simulink model "vocoder_model"  (R2017b)
settings: Solver=VariableStepAuto  StartTime=0.0  StopTime=20  RelTol=1e-3
undefined symbols (not defined in the file or in its folder): NB
libraries: xbsIndex_r4 x1026, dspsrcs4 x1
(part 1 of 8)
settings Model: Creator=8183302  LastModifiedBy=8183302

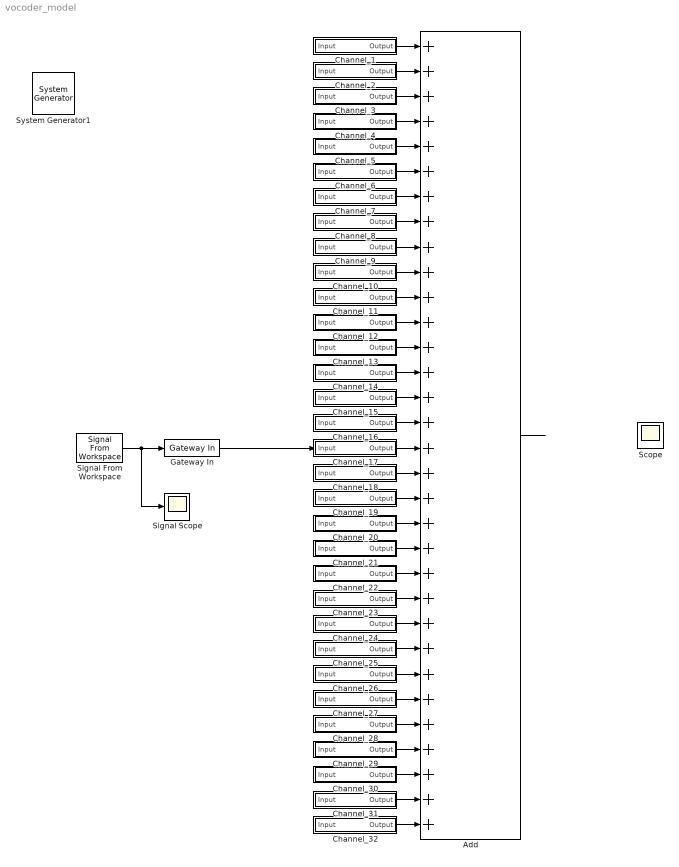
== system vocoder_model ==
  " System Generator1" : xbsIndex_r4/ System Generator  Tag=genX  xilinxfamily=kintex7  part=xc7k325t  speed=-3  package=fbg676  synthesis_tool=Vivado  clock_wrapper=Clock Enables  directory=./netlist  proj_type=Vivado  Synth_file=Vivado Synthesis Defaults  Impl_file=Vivado Implementation Defaults  testbench=off  simulink_period=1/8000  sysclk_period=10  dcm_input_clock_period=10  incr_netlist=off  trim_vbits=Everywhere in SubSystem  dbl_ovrd=According to Block Masks  core_generation=According to Block Masks  run_coregen=off  deprecated_control=off  eval_field=0  block_type=sysgen
  Add : Sum  Inputs=++++++++++++++++++++++++++++++++
  Channel_1 : Subsystem  mask{b0=0.1426970149, b1=0.0000000000, b2=-0.1426970149, a1=-1.6901715989, a2=0.7146059702, fc=299.991723}
  Channel_10 : Subsystem  mask{b0=0.0872963307, b1=0.0000000000, b2=-0.0872963307, a1=-1.4690457093, a2=0.8254073387, fc=816.949484}
  Channel_11 : Subsystem  mask{b0=0.0845435910, b1=0.0000000000, b2=-0.0845435910, a1=-1.4085768543, a2=0.8309128181, fc=888.837275}
  Channel_12 : Subsystem  mask{b0=0.0820880005, b1=0.0000000000, b2=-0.0820880005, a1=-1.3394973368, a2=0.8358239989, fc=964.131808}
  Channel_13 : Subsystem  mask{b0=0.0798861132, b1=0.0000000000, b2=-0.0798861132, a1=-1.2612912570, a2=0.8402277736, fc=1042.994526}
  Channel_14 : Subsystem  mask{b0=0.0779025394, b1=0.0000000000, b2=-0.0779025394, a1=-1.1734445637, a2=0.8441949212, fc=1125.594525}
  Channel_15 : Subsystem  mask{b0=0.0761081589, b1=0.0000000000, b2=-0.0761081589, a1=-1.0754648676, a2=0.8477836822, fc=1212.108914}
  Channel_16 : Subsystem  mask{b0=0.0744787896, b1=0.0000000000, b2=-0.0744787896, a1=-0.9669048108, a2=0.8510424209, fc=1302.723195}
  Channel_17 : Subsystem  mask{b0=0.0729941817, b1=0.0000000000, b2=-0.0729941817, a1=-0.8473898380, a2=0.8540116366, fc=1397.631659}
  Channel_18 : Subsystem  mask{b0=0.0716372491, b1=0.0000000000, b2=-0.0716372491, a1=-0.7166511718, a2=0.8567255018, fc=1497.037808}
  Channel_19 : Subsystem  mask{b0=0.0703934733, b1=0.0000000000, b2=-0.0703934733, a1=-0.5745647402, a2=0.8592130535, fc=1601.154785}
  Channel_2 : Subsystem  mask{b0=0.1312430755, b1=0.0000000000, b2=-0.1312430755, a1=-1.6922316836, a2=0.7375138489, fc=347.381037}
  Channel_20 : Subsystem  mask{b0=0.0692504382, b1=0.0000000000, b2=-0.0692504382, a1=-0.4211967011, a2=0.8614991237, fc=1710.205836}
  Channel_21 : Subsystem  mask{b0=0.0681974623, b1=0.0000000000, b2=-0.0681974623, a1=-0.2568560434, a2=0.8636050755, fc=1824.424783}
  Channel_22 : Subsystem  mask{b0=0.0672253054, b1=0.0000000000, b2=-0.0672253054, a1=-0.0821544768, a2=0.8655493893, fc=1944.056533}
  Channel_23 : Subsystem  mask{b0=0.0663259331, b1=0.0000000000, b2=-0.0663259331, a1=0.1019265783, a2=0.8673481338, fc=2069.357596}
  Channel_24 : Subsystem  mask{b0=0.0654923262, b1=0.0000000000, b2=-0.0654923262, a1=0.2939626743, a2=0.8690153475, fc=2200.596640}
  Channel_25 : Subsystem  mask{b0=0.0647183248, b1=0.0000000000, b2=-0.0647183248, a1=0.4920082741, a2=0.8705633504, fc=2338.055064}
  Channel_26 : Subsystem  mask{b0=0.0639985006, b1=0.0000000000, b2=-0.0639985006, a1=0.6935166168, a2=0.8720029989, fc=2482.027602}
  Channel_27 : Subsystem  mask{b0=0.0633280511, b1=0.0000000000, b2=-0.0633280511, a1=0.8952616127, a2=0.8733438978, fc=2632.822957}
  Channel_28 : Subsystem  mask{b0=0.0627027123, b1=0.0000000000, b2=-0.0627027123, a1=1.0932676802, a2=0.8745945754, fc=2790.764459}
  Channel_29 : Subsystem  mask{b0=0.0621186846, b1=0.0000000000, b2=-0.0621186846, a1=1.2827556587, a2=0.8757626308, fc=2956.190763}
  Channel_3 : Subsystem  mask{b0=0.1219971552, b1=0.0000000000, b2=-0.1219971552, a1=-1.6873845160, a2=0.7560056896, fc=397.016117}
  Channel_30 : Subsystem  mask{b0=0.0615725716, b1=0.0000000000, b2=-0.0615725716, a1=1.4581155660, a2=0.8768548568, fc=3129.456570}
  Channel_31 : Subsystem  mask{b0=0.0610613278, b1=0.0000000000, b2=-0.0610613278, a1=1.6129199398, a2=0.8778773445, fc=3310.933394}
  Channel_32 : Subsystem  mask{b0=0.0605822143, b1=0.0000000000, b2=-0.0605822143, a1=1.7399946660, a2=0.8788355715, fc=3501.010351}
  Channel_4 : Subsystem  mask{b0=0.1143823509, b1=0.0000000000, b2=-0.1143823509, a1=-1.6760436191, a2=0.7712352982, fc=449.003389}
  Channel_5 : Subsystem  mask{b0=0.1080071943, b1=0.0000000000, b2=-0.1080071943, a1=-1.6583545791, a2=0.7839856114, fc=503.454323}
  Channel_6 : Subsystem  mask{b0=0.1025964806, b1=0.0000000000, b2=-0.1025964806, a1=-1.6342751055, a2=0.7948070389, fc=560.485670}
  Channel_7 : Subsystem  mask{b0=0.0979509870, b1=0.0000000000, b2=-0.0979509870, a1=-1.6036256537, a2=0.8040980260, fc=620.219716}
  Channel_8 : Subsystem  mask{b0=0.0939228891, b1=0.0000000000, b2=-0.0939228891, a1=-1.5661230792, a2=0.8121542217, fc=682.784541}
  Channel_9 : Subsystem  mask{b0=0.0904001591, b1=0.0000000000, b2=-0.0904001591, a1=-1.5214045021, a2=0.8191996818, fc=748.314295}
  Gateway In : xbsIndex_r4/Gateway In  gui_display_data_type=Fixed-point  arith_type="Signed  (2's comp)"  n_bits=16  bin_pt=15  preci_type=Single  exp_width=8  frac_width=24  rows=1  columns=1  quantization="Round  (unbiased: +/- Inf)"  overflow=Saturate  period=1/8000  UseAsADC=off  ADCChannel='1'  interface=None  automatic_assignment=on  address_offset=hex2dec('00')  intf_name=''  intf_description=''  default_value=0  timing_constraint=None  locs_specified=off  LOCs={}  io_standard={}  inherit_from_input=off  hdl_port=on  dbl_ovrd=off  block_type=gatewayin
  Scope : Scope
  Signal From Workspace : dspsrcs4/Signal From Workspace  X=x  Ts=1/8000  nsamps=1  OutputAfterFinalValue=Setting to zero  ignoreOrWarnInputAndFrameLengths=off  OutputFrames=off
  Signal Scope : Scope
  wires:
  Signal From Workspace/1 -> Signal Scope/1, Gateway In/1
  Channel_1/1(Output) -> Add/1
  Channel_2/1(Output) -> Add/2
  Channel_3/1(Output) -> Add/3
  Channel_4/1(Output) -> Add/4
  Channel_5/1(Output) -> Add/5
  Channel_6/1(Output) -> Add/6
  Channel_7/1(Output) -> Add/7
  Channel_8/1(Output) -> Add/8
  Channel_9/1(Output) -> Add/9
  Channel_10/1(Output) -> Add/10
  Channel_11/1(Output) -> Add/11
  Channel_12/1(Output) -> Add/12
  Channel_13/1(Output) -> Add/13
  Channel_14/1(Output) -> Add/14
  Channel_15/1(Output) -> Add/15
  Channel_16/1(Output) -> Add/16
  Channel_17/1(Output) -> Add/17
  Channel_18/1(Output) -> Add/18
  Channel_19/1(Output) -> Add/19
  Channel_20/1(Output) -> Add/20
  Channel_21/1(Output) -> Add/21
  Channel_22/1(Output) -> Add/22
  Channel_23/1(Output) -> Add/23
  Channel_24/1(Output) -> Add/24
  Channel_25/1(Output) -> Add/25
  Channel_26/1(Output) -> Add/26
  Channel_27/1(Output) -> Add/27
  Channel_28/1(Output) -> Add/28
  Channel_29/1(Output) -> Add/29
  Channel_30/1(Output) -> Add/30
  Channel_31/1(Output) -> Add/31
  Channel_32/1(Output) -> Add/32
  Add/1 -> ?
  Gateway In/1 -> Channel_17/1(Input)
  ? -> Scope/1

== system vocoder_model/Channel_1 ==
  Input : Inport
  Abs Scope : Scope
  Absolute : xbsIndex_r4/Absolute  precision=User Defined  arith_type="Signed  (2's comp)"  n_bits=16  bin_pt=15  quantization=Truncate  overflow=Wrap  en=off  latency=0  dbl_ovrd=off  block_type=abs
  Convert : xbsIndex_r4/Convert  gui_display_data_type=Fixed-point  arith_type="Signed  (2's comp)"  n_bits=16  bin_pt=15  float_type=Single  exp_bits=8  fraction_bits=24  quantization=Truncate  overflow=Wrap  en=off  latency=0  pipeline=off  dbl_ovrd=off  block_type=convert
  Final Channel Scope : Scope
  Gateway In : xbsIndex_r4/Gateway In  gui_display_data_type=Fixed-point  arith_type="Signed  (2's comp)"  n_bits=16  bin_pt=15  preci_type=Single  exp_width=8  frac_width=24  rows=1  columns=1  quantization=Truncate  overflow=Wrap  period=1/8000  UseAsADC=off  ADCChannel='1'  interface=None  automatic_assignment=on  address_offset=hex2dec('00')  intf_name=''  intf_description=''  default_value=0  timing_constraint=None  locs_specified=off  LOCs={}  io_standard={}  inherit_from_input=off  hdl_port=on  dbl_ovrd=off  block_type=gatewayin
  Gateway Out{,1..3} (4 alike) : xbsIndex_r4/Gateway Out  inherit_from_input=off  hdl_port=off  rows=1  columns=1  UseAsDAC=off  DACChannel='1'  interface=None  automatic_assignment=on  address_offset=hex2dec('00')  intf_name=''  intf_description=''  timing_constraint=None  locs_specified=off  LOCs={}  io_standard={}  block_type=gatewayout
  IIR Filter : Subsystem
  IIR Filter Scope : Scope
  LPF Scope : Scope
  Low Pass Filter : Subsystem
  Mult : xbsIndex_r4/Mult  precision=User Defined  arith_type="Signed  (2's comp)"  n_bits=16  bin_pt=15  quantization=Truncate  overflow=Wrap  en=off  latency=0  use_behavioral_HDL=off  opt=Speed  use_embedded=on  optimum_pipeline=off  pipeline=on  dbl_ovrd=off  use_rpm=on  placement_style=Triangular  block_type=mult
  Sine Wave : Sin  Frequency=2*pi*fc  SampleTime=1/8000
  Output : Outport
  wires:
  Input/1 -> IIR Filter/1(Input)
  IIR Filter/1(Output) -> Gateway Out1/1, Absolute/1
  Sine Wave/1 -> Gateway In/1
  Convert/1 -> Mult/1
  Gateway In/1 -> Mult/2
  Absolute/1 -> Gateway Out2/1, Low Pass Filter/1(Input1)
  Low Pass Filter/1(Output1) -> Gateway Out3/1, Convert/1
  Gateway Out/1 -> Output/1, Final Channel Scope/1
  Mult/1 -> Gateway Out/1
  Gateway Out1/1 -> IIR Filter Scope/1
  Gateway Out2/1 -> Abs Scope/1
  Gateway Out3/1 -> LPF Scope/1

== system vocoder_model/Channel_10 ==
  Input : Inport
  Abs Scope : Scope
  Absolute : xbsIndex_r4/Absolute  precision=User Defined  arith_type="Signed  (2's comp)"  n_bits=16  bin_pt=15  quantization=Truncate  overflow=Wrap  en=off  latency=0  dbl_ovrd=off  block_type=abs
  Convert : xbsIndex_r4/Convert  gui_display_data_type=Fixed-point  arith_type="Signed  (2's comp)"  n_bits=16  bin_pt=15  float_type=Single  exp_bits=8  fraction_bits=24  quantization=Truncate  overflow=Wrap  en=off  latency=0  pipeline=off  dbl_ovrd=off  block_type=convert
  Final Channel Scope : Scope
  Gateway In : xbsIndex_r4/Gateway In  gui_display_data_type=Fixed-point  arith_type="Signed  (2's comp)"  n_bits=16  bin_pt=15  preci_type=Single  exp_width=8  frac_width=24  rows=1  columns=1  quantization=Truncate  overflow=Wrap  period=1/8000  UseAsADC=off  ADCChannel='1'  interface=None  automatic_assignment=on  address_offset=hex2dec('00')  intf_name=''  intf_description=''  default_value=0  timing_constraint=None  locs_specified=off  LOCs={}  io_standard={}  inherit_from_input=off  hdl_port=on  dbl_ovrd=off  block_type=gatewayin
  Gateway Out{,1..3} (4 alike) : xbsIndex_r4/Gateway Out  inherit_from_input=off  hdl_port=off  rows=1  columns=1  UseAsDAC=off  DACChannel='1'  interface=None  automatic_assignment=on  address_offset=hex2dec('00')  intf_name=''  intf_description=''  timing_constraint=None  locs_specified=off  LOCs={}  io_standard={}  block_type=gatewayout
  IIR Filter : Subsystem
  IIR Filter Scope : Scope
  LPF Scope : Scope
  Low Pass Filter : Subsystem
  Mult : xbsIndex_r4/Mult  precision=User Defined  arith_type="Signed  (2's comp)"  n_bits=16  bin_pt=15  quantization=Truncate  overflow=Wrap  en=off  latency=0  use_behavioral_HDL=off  opt=Speed  use_embedded=on  optimum_pipeline=off  pipeline=on  dbl_ovrd=off  use_rpm=on  placement_style=Triangular  block_type=mult
  Sine Wave : Sin  Frequency=2*pi*fc  SampleTime=1/8000
  Output : Outport
  wires:
  Input/1 -> IIR Filter/1(Input)
  IIR Filter/1(Output) -> Gateway Out1/1, Absolute/1
  Sine Wave/1 -> Gateway In/1
  Convert/1 -> Mult/1
  Gateway In/1 -> Mult/2
  Absolute/1 -> Gateway Out2/1, Low Pass Filter/1(Input1)
  Low Pass Filter/1(Output1) -> Gateway Out3/1, Convert/1
  Gateway Out/1 -> Output/1, Final Channel Scope/1
  Mult/1 -> Gateway Out/1
  Gateway Out1/1 -> IIR Filter Scope/1
  Gateway Out2/1 -> Abs Scope/1
  Gateway Out3/1 -> LPF Scope/1

== system vocoder_model/Channel_11 ==
  Input : Inport
  Abs Scope : Scope
  Absolute : xbsIndex_r4/Absolute  precision=User Defined  arith_type="Signed  (2's comp)"  n_bits=16  bin_pt=15  quantization=Truncate  overflow=Wrap  en=off  latency=0  dbl_ovrd=off  block_type=abs
  Convert : xbsIndex_r4/Convert  gui_display_data_type=Fixed-point  arith_type="Signed  (2's comp)"  n_bits=16  bin_pt=15  float_type=Single  exp_bits=8  fraction_bits=24  quantization=Truncate  overflow=Wrap  en=off  latency=0  pipeline=off  dbl_ovrd=off  block_type=convert
  Final Channel Scope : Scope
  Gateway In : xbsIndex_r4/Gateway In  gui_display_data_type=Fixed-point  arith_type="Signed  (2's comp)"  n_bits=16  bin_pt=15  preci_type=Single  exp_width=8  frac_width=24  rows=1  columns=1  quantization=Truncate  overflow=Wrap  period=1/8000  UseAsADC=off  ADCChannel='1'  interface=None  automatic_assignment=on  address_offset=hex2dec('00')  intf_name=''  intf_description=''  default_value=0  timing_constraint=None  locs_specified=off  LOCs={}  io_standard={}  inherit_from_input=off  hdl_port=on  dbl_ovrd=off  block_type=gatewayin
  Gateway Out{,1..3} (4 alike) : xbsIndex_r4/Gateway Out  inherit_from_input=off  hdl_port=off  rows=1  columns=1  UseAsDAC=off  DACChannel='1'  interface=None  automatic_assignment=on  address_offset=hex2dec('00')  intf_name=''  intf_description=''  timing_constraint=None  locs_specified=off  LOCs={}  io_standard={}  block_type=gatewayout
  IIR Filter : Subsystem
  IIR Filter Scope : Scope
  LPF Scope : Scope
  Low Pass Filter : Subsystem
  Mult : xbsIndex_r4/Mult  precision=User Defined  arith_type="Signed  (2's comp)"  n_bits=16  bin_pt=15  quantization=Truncate  overflow=Wrap  en=off  latency=0  use_behavioral_HDL=off  opt=Speed  use_embedded=on  optimum_pipeline=off  pipeline=on  dbl_ovrd=off  use_rpm=on  placement_style=Triangular  block_type=mult
  Sine Wave : Sin  Frequency=2*pi*fc  SampleTime=1/8000
  Output : Outport
  wires:
  Input/1 -> IIR Filter/1(Input)
  IIR Filter/1(Output) -> Gateway Out1/1, Absolute/1
  Sine Wave/1 -> Gateway In/1
  Convert/1 -> Mult/1
  Gateway In/1 -> Mult/2
  Absolute/1 -> Gateway Out2/1, Low Pass Filter/1(Input1)
  Low Pass Filter/1(Output1) -> Gateway Out3/1, Convert/1
  Gateway Out/1 -> Output/1, Final Channel Scope/1
  Mult/1 -> Gateway Out/1
  Gateway Out1/1 -> IIR Filter Scope/1
  Gateway Out2/1 -> Abs Scope/1
  Gateway Out3/1 -> LPF Scope/1

== system vocoder_model/Channel_12 ==
  Input : Inport
  Abs Scope : Scope
  Absolute : xbsIndex_r4/Absolute  precision=User Defined  arith_type="Signed  (2's comp)"  n_bits=16  bin_pt=15  quantization=Truncate  overflow=Wrap  en=off  latency=0  dbl_ovrd=off  block_type=abs
  Convert : xbsIndex_r4/Convert  gui_display_data_type=Fixed-point  arith_type="Signed  (2's comp)"  n_bits=16  bin_pt=15  float_type=Single  exp_bits=8  fraction_bits=24  quantization=Truncate  overflow=Wrap  en=off  latency=0  pipeline=off  dbl_ovrd=off  block_type=convert
  Final Channel Scope : Scope
  Gateway In : xbsIndex_r4/Gateway In  gui_display_data_type=Fixed-point  arith_type="Signed  (2's comp)"  n_bits=16  bin_pt=15  preci_type=Single  exp_width=8  frac_width=24  rows=1  columns=1  quantization=Truncate  overflow=Wrap  period=1/8000  UseAsADC=off  ADCChannel='1'  interface=None  automatic_assignment=on  address_offset=hex2dec('00')  intf_name=''  intf_description=''  default_value=0  timing_constraint=None  locs_specified=off  LOCs={}  io_standard={}  inherit_from_input=off  hdl_port=on  dbl_ovrd=off  block_type=gatewayin
  Gateway Out{,1..3} (4 alike) : xbsIndex_r4/Gateway Out  inherit_from_input=off  hdl_port=off  rows=1  columns=1  UseAsDAC=off  DACChannel='1'  interface=None  automatic_assignment=on  address_offset=hex2dec('00')  intf_name=''  intf_description=''  timing_constraint=None  locs_specified=off  LOCs={}  io_standard={}  block_type=gatewayout
  IIR Filter : Subsystem
  IIR Filter Scope : Scope
  LPF Scope : Scope
  Low Pass Filter : Subsystem
  Mult : xbsIndex_r4/Mult  precision=User Defined  arith_type="Signed  (2's comp)"  n_bits=16  bin_pt=15  quantization=Truncate  overflow=Wrap  en=off  latency=0  use_behavioral_HDL=off  opt=Speed  use_embedded=on  optimum_pipeline=off  pipeline=on  dbl_ovrd=off  use_rpm=on  placement_style=Triangular  block_type=mult
  Sine Wave : Sin  Frequency=2*pi*fc  SampleTime=1/8000
  Output : Outport
  wires:
  Input/1 -> IIR Filter/1(Input)
  IIR Filter/1(Output) -> Gateway Out1/1, Absolute/1
  Sine Wave/1 -> Gateway In/1
  Convert/1 -> Mult/1
  Gateway In/1 -> Mult/2
  Absolute/1 -> Gateway Out2/1, Low Pass Filter/1(Input1)
  Low Pass Filter/1(Output1) -> Gateway Out3/1, Convert/1
  Gateway Out/1 -> Output/1, Final Channel Scope/1
  Mult/1 -> Gateway Out/1
  Gateway Out1/1 -> IIR Filter Scope/1
  Gateway Out2/1 -> Abs Scope/1
  Gateway Out3/1 -> LPF Scope/1

== system vocoder_model/Channel_13 ==
  Input : Inport
  Abs Scope : Scope
  Absolute : xbsIndex_r4/Absolute  precision=User Defined  arith_type="Signed  (2's comp)"  n_bits=16  bin_pt=15  quantization=Truncate  overflow=Wrap  en=off  latency=0  dbl_ovrd=off  block_type=abs
  Convert : xbsIndex_r4/Convert  gui_display_data_type=Fixed-point  arith_type="Signed  (2's comp)"  n_bits=16  bin_pt=15  float_type=Single  exp_bits=8  fraction_bits=24  quantization=Truncate  overflow=Wrap  en=off  latency=0  pipeline=off  dbl_ovrd=off  block_type=convert
  Final Channel Scope : Scope
  Gateway In : xbsIndex_r4/Gateway In  gui_display_data_type=Fixed-point  arith_type="Signed  (2's comp)"  n_bits=16  bin_pt=15  preci_type=Single  exp_width=8  frac_width=24  rows=1  columns=1  quantization=Truncate  overflow=Wrap  period=1/8000  UseAsADC=off  ADCChannel='1'  interface=None  automatic_assignment=on  address_offset=hex2dec('00')  intf_name=''  intf_description=''  default_value=0  timing_constraint=None  locs_specified=off  LOCs={}  io_standard={}  inherit_from_input=off  hdl_port=on  dbl_ovrd=off  block_type=gatewayin
  Gateway Out{,1..3} (4 alike) : xbsIndex_r4/Gateway Out  inherit_from_input=off  hdl_port=off  rows=1  columns=1  UseAsDAC=off  DACChannel='1'  interface=None  automatic_assignment=on  address_offset=hex2dec('00')  intf_name=''  intf_description=''  timing_constraint=None  locs_specified=off  LOCs={}  io_standard={}  block_type=gatewayout
  IIR Filter : Subsystem
  IIR Filter Scope : Scope
  LPF Scope : Scope
  Low Pass Filter : Subsystem
  Mult : xbsIndex_r4/Mult  precision=User Defined  arith_type="Signed  (2's comp)"  n_bits=16  bin_pt=15  quantization=Truncate  overflow=Wrap  en=off  latency=0  use_behavioral_HDL=off  opt=Speed  use_embedded=on  optimum_pipeline=off  pipeline=on  dbl_ovrd=off  use_rpm=on  placement_style=Triangular  block_type=mult
  Sine Wave : Sin  Frequency=2*pi*fc  SampleTime=1/8000
  Output : Outport
  wires:
  Input/1 -> IIR Filter/1(Input)
  IIR Filter/1(Output) -> Gateway Out1/1, Absolute/1
  Sine Wave/1 -> Gateway In/1
  Convert/1 -> Mult/1
  Gateway In/1 -> Mult/2
  Absolute/1 -> Gateway Out2/1, Low Pass Filter/1(Input1)
  Low Pass Filter/1(Output1) -> Gateway Out3/1, Convert/1
  Gateway Out/1 -> Output/1, Final Channel Scope/1
  Mult/1 -> Gateway Out/1
  Gateway Out1/1 -> IIR Filter Scope/1
  Gateway Out2/1 -> Abs Scope/1
  Gateway Out3/1 -> LPF Scope/1

== system vocoder_model/Channel_14 ==
  Input : Inport
  Abs Scope : Scope
  Absolute : xbsIndex_r4/Absolute  precision=User Defined  arith_type="Signed  (2's comp)"  n_bits=16  bin_pt=15  quantization=Truncate  overflow=Wrap  en=off  latency=0  dbl_ovrd=off  block_type=abs
  Convert : xbsIndex_r4/Convert  gui_display_data_type=Fixed-point  arith_type="Signed  (2's comp)"  n_bits=16  bin_pt=15  float_type=Single  exp_bits=8  fraction_bits=24  quantization=Truncate  overflow=Wrap  en=off  latency=0  pipeline=off  dbl_ovrd=off  block_type=convert
  Final Channel Scope : Scope
  Gateway In : xbsIndex_r4/Gateway In  gui_display_data_type=Fixed-point  arith_type="Signed  (2's comp)"  n_bits=16  bin_pt=15  preci_type=Single  exp_width=8  frac_width=24  rows=1  columns=1  quantization=Truncate  overflow=Wrap  period=1/8000  UseAsADC=off  ADCChannel='1'  interface=None  automatic_assignment=on  address_offset=hex2dec('00')  intf_name=''  intf_description=''  default_value=0  timing_constraint=None  locs_specified=off  LOCs={}  io_standard={}  inherit_from_input=off  hdl_port=on  dbl_ovrd=off  block_type=gatewayin
  Gateway Out{,1..3} (4 alike) : xbsIndex_r4/Gateway Out  inherit_from_input=off  hdl_port=off  rows=1  columns=1  UseAsDAC=off  DACChannel='1'  interface=None  automatic_assignment=on  address_offset=hex2dec('00')  intf_name=''  intf_description=''  timing_constraint=None  locs_specified=off  LOCs={}  io_standard={}  block_type=gatewayout
  IIR Filter : Subsystem
  IIR Filter Scope : Scope
  LPF Scope : Scope
  Low Pass Filter : Subsystem
  Mult : xbsIndex_r4/Mult  precision=User Defined  arith_type="Signed  (2's comp)"  n_bits=16  bin_pt=15  quantization=Truncate  overflow=Wrap  en=off  latency=0  use_behavioral_HDL=off  opt=Speed  use_embedded=on  optimum_pipeline=off  pipeline=on  dbl_ovrd=off  use_rpm=on  placement_style=Triangular  block_type=mult
  Sine Wave : Sin  Frequency=2*pi*fc  SampleTime=1/8000
  Output : Outport
  wires:
  Input/1 -> IIR Filter/1(Input)
  IIR Filter/1(Output) -> Gateway Out1/1, Absolute/1
  Sine Wave/1 -> Gateway In/1
  Convert/1 -> Mult/1
  Gateway In/1 -> Mult/2
  Absolute/1 -> Gateway Out2/1, Low Pass Filter/1(Input1)
  Low Pass Filter/1(Output1) -> Gateway Out3/1, Convert/1
  Gateway Out/1 -> Output/1, Final Channel Scope/1
  Mult/1 -> Gateway Out/1
  Gateway Out1/1 -> IIR Filter Scope/1
  Gateway Out2/1 -> Abs Scope/1
  Gateway Out3/1 -> LPF Scope/1

== system vocoder_model/Channel_15 ==
  Input : Inport
  Abs Scope : Scope
  Absolute : xbsIndex_r4/Absolute  precision=User Defined  arith_type="Signed  (2's comp)"  n_bits=16  bin_pt=15  quantization=Truncate  overflow=Wrap  en=off  latency=0  dbl_ovrd=off  block_type=abs
  Convert : xbsIndex_r4/Convert  gui_display_data_type=Fixed-point  arith_type="Signed  (2's comp)"  n_bits=16  bin_pt=15  float_type=Single  exp_bits=8  fraction_bits=24  quantization=Truncate  overflow=Wrap  en=off  latency=0  pipeline=off  dbl_ovrd=off  block_type=convert
  Final Channel Scope : Scope
  Gateway In : xbsIndex_r4/Gateway In  gui_display_data_type=Fixed-point  arith_type="Signed  (2's comp)"  n_bits=16  bin_pt=15  preci_type=Single  exp_width=8  frac_width=24  rows=1  columns=1  quantization=Truncate  overflow=Wrap  period=1/8000  UseAsADC=off  ADCChannel='1'  interface=None  automatic_assignment=on  address_offset=hex2dec('00')  intf_name=''  intf_description=''  default_value=0  timing_constraint=None  locs_specified=off  LOCs={}  io_standard={}  inherit_from_input=off  hdl_port=on  dbl_ovrd=off  block_type=gatewayin
  Gateway Out{,1..3} (4 alike) : xbsIndex_r4/Gateway Out  inherit_from_input=off  hdl_port=off  rows=1  columns=1  UseAsDAC=off  DACChannel='1'  interface=None  automatic_assignment=on  address_offset=hex2dec('00')  intf_name=''  intf_description=''  timing_constraint=None  locs_specified=off  LOCs={}  io_standard={}  block_type=gatewayout
  IIR Filter : Subsystem
  IIR Filter Scope : Scope
  LPF Scope : Scope
  Low Pass Filter : Subsystem
  Mult : xbsIndex_r4/Mult  precision=User Defined  arith_type="Signed  (2's comp)"  n_bits=16  bin_pt=15  quantization=Truncate  overflow=Wrap  en=off  latency=0  use_behavioral_HDL=off  opt=Speed  use_embedded=on  optimum_pipeline=off  pipeline=on  dbl_ovrd=off  use_rpm=on  placement_style=Triangular  block_type=mult
  Sine Wave : Sin  Frequency=2*pi*fc  SampleTime=1/8000
  Output : Outport
  wires:
  Input/1 -> IIR Filter/1(Input)
  IIR Filter/1(Output) -> Gateway Out1/1, Absolute/1
  Sine Wave/1 -> Gateway In/1
  Convert/1 -> Mult/1
  Gateway In/1 -> Mult/2
  Absolute/1 -> Gateway Out2/1, Low Pass Filter/1(Input1)
  Low Pass Filter/1(Output1) -> Gateway Out3/1, Convert/1
  Gateway Out/1 -> Output/1, Final Channel Scope/1
  Mult/1 -> Gateway Out/1
  Gateway Out1/1 -> IIR Filter Scope/1
  Gateway Out2/1 -> Abs Scope/1
  Gateway Out3/1 -> LPF Scope/1

== system vocoder_model/Channel_16 ==
  Input : Inport
  Abs Scope : Scope
  Absolute : xbsIndex_r4/Absolute  precision=User Defined  arith_type="Signed  (2's comp)"  n_bits=16  bin_pt=15  quantization=Truncate  overflow=Wrap  en=off  latency=0  dbl_ovrd=off  block_type=abs
  Convert : xbsIndex_r4/Convert  gui_display_data_type=Fixed-point  arith_type="Signed  (2's comp)"  n_bits=16  bin_pt=15  float_type=Single  exp_bits=8  fraction_bits=24  quantization=Truncate  overflow=Wrap  en=off  latency=0  pipeline=off  dbl_ovrd=off  block_type=convert
  Final Channel Scope : Scope
  Gateway In : xbsIndex_r4/Gateway In  gui_display_data_type=Fixed-point  arith_type="Signed  (2's comp)"  n_bits=16  bin_pt=15  preci_type=Single  exp_width=8  frac_width=24  rows=1  columns=1  quantization=Truncate  overflow=Wrap  period=1/8000  UseAsADC=off  ADCChannel='1'  interface=None  automatic_assignment=on  address_offset=hex2dec('00')  intf_name=''  intf_description=''  default_value=0  timing_constraint=None  locs_specified=off  LOCs={}  io_standard={}  inherit_from_input=off  hdl_port=on  dbl_ovrd=off  block_type=gatewayin
  Gateway Out{,1..3} (4 alike) : xbsIndex_r4/Gateway Out  inherit_from_input=off  hdl_port=off  rows=1  columns=1  UseAsDAC=off  DACChannel='1'  interface=None  automatic_assignment=on  address_offset=hex2dec('00')  intf_name=''  intf_description=''  timing_constraint=None  locs_specified=off  LOCs={}  io_standard={}  block_type=gatewayout
  IIR Filter : Subsystem
  IIR Filter Scope : Scope
  LPF Scope : Scope
  Low Pass Filter : Subsystem
  Mult : xbsIndex_r4/Mult  precision=User Defined  arith_type="Signed  (2's comp)"  n_bits=16  bin_pt=15  quantization=Truncate  overflow=Wrap  en=off  latency=0  use_behavioral_HDL=off  opt=Speed  use_embedded=on  optimum_pipeline=off  pipeline=on  dbl_ovrd=off  use_rpm=on  placement_style=Triangular  block_type=mult
  Sine Wave : Sin  Frequency=2*pi*fc  SampleTime=1/8000
  Output : Outport
  wires:
  Input/1 -> IIR Filter/1(Input)
  IIR Filter/1(Output) -> Gateway Out1/1, Absolute/1
  Sine Wave/1 -> Gateway In/1
  Convert/1 -> Mult/1
  Gateway In/1 -> Mult/2
  Absolute/1 -> Gateway Out2/1, Low Pass Filter/1(Input1)
  Low Pass Filter/1(Output1) -> Gateway Out3/1, Convert/1
  Gateway Out/1 -> Output/1, Final Channel Scope/1
  Mult/1 -> Gateway Out/1
  Gateway Out1/1 -> IIR Filter Scope/1
  Gateway Out2/1 -> Abs Scope/1
  Gateway Out3/1 -> LPF Scope/1

== system vocoder_model/Channel_17 ==
  Input : Inport
  Abs Scope : Scope
  Absolute : xbsIndex_r4/Absolute  precision=User Defined  arith_type="Signed  (2's comp)"  n_bits=16  bin_pt=15  quantization=Truncate  overflow=Wrap  en=off  latency=0  dbl_ovrd=off  block_type=abs
  Convert : xbsIndex_r4/Convert  gui_display_data_type=Fixed-point  arith_type="Signed  (2's comp)"  n_bits=16  bin_pt=15  float_type=Single  exp_bits=8  fraction_bits=24  quantization=Truncate  overflow=Wrap  en=off  latency=0  pipeline=off  dbl_ovrd=off  block_type=convert
  Final Channel Scope : Scope
  Gateway In : xbsIndex_r4/Gateway In  gui_display_data_type=Fixed-point  arith_type="Signed  (2's comp)"  n_bits=16  bin_pt=15  preci_type=Single  exp_width=8  frac_width=24  rows=1  columns=1  quantization=Truncate  overflow=Wrap  period=1/8000  UseAsADC=off  ADCChannel='1'  interface=None  automatic_assignment=on  address_offset=hex2dec('00')  intf_name=''  intf_description=''  default_value=0  timing_constraint=None  locs_specified=off  LOCs={}  io_standard={}  inherit_from_input=off  hdl_port=on  dbl_ovrd=off  block_type=gatewayin
  Gateway Out{,1..3} (4 alike) : xbsIndex_r4/Gateway Out  inherit_from_input=off  hdl_port=off  rows=1  columns=1  UseAsDAC=off  DACChannel='1'  interface=None  automatic_assignment=on  address_offset=hex2dec('00')  intf_name=''  intf_description=''  timing_constraint=None  locs_specified=off  LOCs={}  io_standard={}  block_type=gatewayout
  IIR Filter : Subsystem
  IIR Filter Scope : Scope
  LPF Scope : Scope
  Low Pass Filter : Subsystem
  Mult : xbsIndex_r4/Mult  precision=User Defined  arith_type="Signed  (2's comp)"  n_bits=16  bin_pt=15  quantization=Truncate  overflow=Wrap  en=off  latency=0  use_behavioral_HDL=off  opt=Speed  use_embedded=on  optimum_pipeline=off  pipeline=on  dbl_ovrd=off  use_rpm=on  placement_style=Triangular  block_type=mult
  Sine Wave : Sin  Frequency=2*pi*fc  SampleTime=1/8000
  Output : Outport
  wires:
  Input/1 -> IIR Filter/1(Input)
  IIR Filter/1(Output) -> Gateway Out1/1, Absolute/1
  Sine Wave/1 -> Gateway In/1
  Convert/1 -> Mult/1
  Gateway In/1 -> Mult/2
  Absolute/1 -> Gateway Out2/1, Low Pass Filter/1(Input1)
  Low Pass Filter/1(Output1) -> Gateway Out3/1, Convert/1
  Gateway Out/1 -> Output/1, Final Channel Scope/1
  Mult/1 -> Gateway Out/1
  Gateway Out1/1 -> IIR Filter Scope/1
  Gateway Out2/1 -> Abs Scope/1
  Gateway Out3/1 -> LPF Scope/1

== system vocoder_model/Channel_18 ==
  Input : Inport
  Abs Scope : Scope
  Absolute : xbsIndex_r4/Absolute  precision=User Defined  arith_type="Signed  (2's comp)"  n_bits=16  bin_pt=15  quantization=Truncate  overflow=Wrap  en=off  latency=0  dbl_ovrd=off  block_type=abs
  Convert : xbsIndex_r4/Convert  gui_display_data_type=Fixed-point  arith_type="Signed  (2's comp)"  n_bits=16  bin_pt=15  float_type=Single  exp_bits=8  fraction_bits=24  quantization=Truncate  overflow=Wrap  en=off  latency=0  pipeline=off  dbl_ovrd=off  block_type=convert
  Final Channel Scope : Scope
  Gateway In : xbsIndex_r4/Gateway In  gui_display_data_type=Fixed-point  arith_type="Signed  (2's comp)"  n_bits=16  bin_pt=15  preci_type=Single  exp_width=8  frac_width=24  rows=1  columns=1  quantization=Truncate  overflow=Wrap  period=1/8000  UseAsADC=off  ADCChannel='1'  interface=None  automatic_assignment=on  address_offset=hex2dec('00')  intf_name=''  intf_description=''  default_value=0  timing_constraint=None  locs_specified=off  LOCs={}  io_standard={}  inherit_from_input=off  hdl_port=on  dbl_ovrd=off  block_type=gatewayin
  Gateway Out{,1..3} (4 alike) : xbsIndex_r4/Gateway Out  inherit_from_input=off  hdl_port=off  rows=1  columns=1  UseAsDAC=off  DACChannel='1'  interface=None  automatic_assignment=on  address_offset=hex2dec('00')  intf_name=''  intf_description=''  timing_constraint=None  locs_specified=off  LOCs={}  io_standard={}  block_type=gatewayout
  IIR Filter : Subsystem
  IIR Filter Scope : Scope
  LPF Scope : Scope
  Low Pass Filter : Subsystem
  Mult : xbsIndex_r4/Mult  precision=User Defined  arith_type="Signed  (2's comp)"  n_bits=16  bin_pt=15  quantization=Truncate  overflow=Wrap  en=off  latency=0  use_behavioral_HDL=off  opt=Speed  use_embedded=on  optimum_pipeline=off  pipeline=on  dbl_ovrd=off  use_rpm=on  placement_style=Triangular  block_type=mult
  Sine Wave : Sin  Frequency=2*pi*fc  SampleTime=1/8000
  Output : Outport
  wires:
  Input/1 -> IIR Filter/1(Input)
  IIR Filter/1(Output) -> Gateway Out1/1, Absolute/1
  Sine Wave/1 -> Gateway In/1
  Convert/1 -> Mult/1
  Gateway In/1 -> Mult/2
  Absolute/1 -> Gateway Out2/1, Low Pass Filter/1(Input1)
  Low Pass Filter/1(Output1) -> Gateway Out3/1, Convert/1
  Gateway Out/1 -> Output/1, Final Channel Scope/1
  Mult/1 -> Gateway Out/1
  Gateway Out1/1 -> IIR Filter Scope/1
  Gateway Out2/1 -> Abs Scope/1
  Gateway Out3/1 -> LPF Scope/1

== system vocoder_model/Channel_19 ==
  Input : Inport
  Abs Scope : Scope
  Absolute : xbsIndex_r4/Absolute  precision=User Defined  arith_type="Signed  (2's comp)"  n_bits=16  bin_pt=15  quantization=Truncate  overflow=Wrap  en=off  latency=0  dbl_ovrd=off  block_type=abs
  Convert : xbsIndex_r4/Convert  gui_display_data_type=Fixed-point  arith_type="Signed  (2's comp)"  n_bits=16  bin_pt=15  float_type=Single  exp_bits=8  fraction_bits=24  quantization=Truncate  overflow=Wrap  en=off  latency=0  pipeline=off  dbl_ovrd=off  block_type=convert
  Final Channel Scope : Scope
  Gateway In : xbsIndex_r4/Gateway In  gui_display_data_type=Fixed-point  arith_type="Signed  (2's comp)"  n_bits=16  bin_pt=15  preci_type=Single  exp_width=8  frac_width=24  rows=1  columns=1  quantization=Truncate  overflow=Wrap  period=1/8000  UseAsADC=off  ADCChannel='1'  interface=None  automatic_assignment=on  address_offset=hex2dec('00')  intf_name=''  intf_description=''  default_value=0  timing_constraint=None  locs_specified=off  LOCs={}  io_standard={}  inherit_from_input=off  hdl_port=on  dbl_ovrd=off  block_type=gatewayin
  Gateway Out{,1..3} (4 alike) : xbsIndex_r4/Gateway Out  inherit_from_input=off  hdl_port=off  rows=1  columns=1  UseAsDAC=off  DACChannel='1'  interface=None  automatic_assignment=on  address_offset=hex2dec('00')  intf_name=''  intf_description=''  timing_constraint=None  locs_specified=off  LOCs={}  io_standard={}  block_type=gatewayout
  IIR Filter : Subsystem
  IIR Filter Scope : Scope
  LPF Scope : Scope
  Low Pass Filter : Subsystem
  Mult : xbsIndex_r4/Mult  precision=User Defined  arith_type="Signed  (2's comp)"  n_bits=16  bin_pt=15  quantization=Truncate  overflow=Wrap  en=off  latency=0  use_behavioral_HDL=off  opt=Speed  use_embedded=on  optimum_pipeline=off  pipeline=on  dbl_ovrd=off  use_rpm=on  placement_style=Triangular  block_type=mult
  Sine Wave : Sin  Frequency=2*pi*fc  SampleTime=1/8000
  Output : Outport
  wires:
  Input/1 -> IIR Filter/1(Input)
  IIR Filter/1(Output) -> Gateway Out1/1, Absolute/1
  Sine Wave/1 -> Gateway In/1
  Convert/1 -> Mult/1
  Gateway In/1 -> Mult/2
  Absolute/1 -> Gateway Out2/1, Low Pass Filter/1(Input1)
  Low Pass Filter/1(Output1) -> Gateway Out3/1, Convert/1
  Gateway Out/1 -> Output/1, Final Channel Scope/1
  Mult/1 -> Gateway Out/1
  Gateway Out1/1 -> IIR Filter Scope/1
  Gateway Out2/1 -> Abs Scope/1
  Gateway Out3/1 -> LPF Scope/1

== system vocoder_model/Channel_2 ==
  Input : Inport
  Abs Scope : Scope
  Absolute : xbsIndex_r4/Absolute  precision=User Defined  arith_type="Signed  (2's comp)"  n_bits=16  bin_pt=15  quantization=Truncate  overflow=Wrap  en=off  latency=0  dbl_ovrd=off  block_type=abs
  Convert : xbsIndex_r4/Convert  gui_display_data_type=Fixed-point  arith_type="Signed  (2's comp)"  n_bits=16  bin_pt=15  float_type=Single  exp_bits=8  fraction_bits=24  quantization=Truncate  overflow=Wrap  en=off  latency=0  pipeline=off  dbl_ovrd=off  block_type=convert
  Final Channel Scope : Scope
  Gateway In : xbsIndex_r4/Gateway In  gui_display_data_type=Fixed-point  arith_type="Signed  (2's comp)"  n_bits=16  bin_pt=15  preci_type=Single  exp_width=8  frac_width=24  rows=1  columns=1  quantization=Truncate  overflow=Wrap  period=1/8000  UseAsADC=off  ADCChannel='1'  interface=None  automatic_assignment=on  address_offset=hex2dec('00')  intf_name=''  intf_description=''  default_value=0  timing_constraint=None  locs_specified=off  LOCs={}  io_standard={}  inherit_from_input=off  hdl_port=on  dbl_ovrd=off  block_type=gatewayin
  Gateway Out{,1..3} (4 alike) : xbsIndex_r4/Gateway Out  inherit_from_input=off  hdl_port=off  rows=1  columns=1  UseAsDAC=off  DACChannel='1'  interface=None  automatic_assignment=on  address_offset=hex2dec('00')  intf_name=''  intf_description=''  timing_constraint=None  locs_specified=off  LOCs={}  io_standard={}  block_type=gatewayout
  IIR Filter : Subsystem
  IIR Filter Scope : Scope
  LPF Scope : Scope
  Low Pass Filter : Subsystem
  Mult : xbsIndex_r4/Mult  precision=User Defined  arith_type="Signed  (2's comp)"  n_bits=16  bin_pt=15  quantization=Truncate  overflow=Wrap  en=off  latency=0  use_behavioral_HDL=off  opt=Speed  use_embedded=on  optimum_pipeline=off  pipeline=on  dbl_ovrd=off  use_rpm=on  placement_style=Triangular  block_type=mult
  Sine Wave : Sin  Frequency=2*pi*fc  SampleTime=1/8000
  Output : Outport
  wires:
  Input/1 -> IIR Filter/1(Input)
  IIR Filter/1(Output) -> Gateway Out1/1, Absolute/1
  Sine Wave/1 -> Gateway In/1
  Convert/1 -> Mult/1
  Gateway In/1 -> Mult/2
  Absolute/1 -> Gateway Out2/1, Low Pass Filter/1(Input1)
  Low Pass Filter/1(Output1) -> Gateway Out3/1, Convert/1
  Gateway Out/1 -> Output/1, Final Channel Scope/1
  Mult/1 -> Gateway Out/1
  Gateway Out1/1 -> IIR Filter Scope/1
  Gateway Out2/1 -> Abs Scope/1
  Gateway Out3/1 -> LPF Scope/1

== system vocoder_model/Channel_20 ==
  Input : Inport
  Abs Scope : Scope
  Absolute : xbsIndex_r4/Absolute  precision=User Defined  arith_type="Signed  (2's comp)"  n_bits=16  bin_pt=15  quantization=Truncate  overflow=Wrap  en=off  latency=0  dbl_ovrd=off  block_type=abs
  Convert : xbsIndex_r4/Convert  gui_display_data_type=Fixed-point  arith_type="Signed  (2's comp)"  n_bits=16  bin_pt=15  float_type=Single  exp_bits=8  fraction_bits=24  quantization=Truncate  overflow=Wrap  en=off  latency=0  pipeline=off  dbl_ovrd=off  block_type=convert
  Final Channel Scope : Scope
  Gateway In : xbsIndex_r4/Gateway In  gui_display_data_type=Fixed-point  arith_type="Signed  (2's comp)"  n_bits=16  bin_pt=15  preci_type=Single  exp_width=8  frac_width=24  rows=1  columns=1  quantization=Truncate  overflow=Wrap  period=1/8000  UseAsADC=off  ADCChannel='1'  interface=None  automatic_assignment=on  address_offset=hex2dec('00')  intf_name=''  intf_description=''  default_value=0  timing_constraint=None  locs_specified=off  LOCs={}  io_standard={}  inherit_from_input=off  hdl_port=on  dbl_ovrd=off  block_type=gatewayin
  Gateway Out{,1..3} (4 alike) : xbsIndex_r4/Gateway Out  inherit_from_input=off  hdl_port=off  rows=1  columns=1  UseAsDAC=off  DACChannel='1'  interface=None  automatic_assignment=on  address_offset=hex2dec('00')  intf_name=''  intf_description=''  timing_constraint=None  locs_specified=off  LOCs={}  io_standard={}  block_type=gatewayout
  IIR Filter : Subsystem
  IIR Filter Scope : Scope
  LPF Scope : Scope
  Low Pass Filter : Subsystem
  Mult : xbsIndex_r4/Mult  precision=User Defined  arith_type="Signed  (2's comp)"  n_bits=16  bin_pt=15  quantization=Truncate  overflow=Wrap  en=off  latency=0  use_behavioral_HDL=off  opt=Speed  use_embedded=on  optimum_pipeline=off  pipeline=on  dbl_ovrd=off  use_rpm=on  placement_style=Triangular  block_type=mult
  Sine Wave : Sin  Frequency=2*pi*fc  SampleTime=1/8000
  Output : Outport
  wires:
  Input/1 -> IIR Filter/1(Input)
  IIR Filter/1(Output) -> Gateway Out1/1, Absolute/1
  Sine Wave/1 -> Gateway In/1
  Convert/1 -> Mult/1
  Gateway In/1 -> Mult/2
  Absolute/1 -> Gateway Out2/1, Low Pass Filter/1(Input1)
  Low Pass Filter/1(Output1) -> Gateway Out3/1, Convert/1
  Gateway Out/1 -> Output/1, Final Channel Scope/1
  Mult/1 -> Gateway Out/1
  Gateway Out1/1 -> IIR Filter Scope/1
  Gateway Out2/1 -> Abs Scope/1
  Gateway Out3/1 -> LPF Scope/1

== system vocoder_model/Channel_21 ==
  Input : Inport
  Abs Scope : Scope
  Absolute : xbsIndex_r4/Absolute  precision=User Defined  arith_type="Signed  (2's comp)"  n_bits=16  bin_pt=15  quantization=Truncate  overflow=Wrap  en=off  latency=0  dbl_ovrd=off  block_type=abs
  Convert : xbsIndex_r4/Convert  gui_display_data_type=Fixed-point  arith_type="Signed  (2's comp)"  n_bits=16  bin_pt=15  float_type=Single  exp_bits=8  fraction_bits=24  quantization=Truncate  overflow=Wrap  en=off  latency=0  pipeline=off  dbl_ovrd=off  block_type=convert
  Final Channel Scope : Scope
  Gateway In : xbsIndex_r4/Gateway In  gui_display_data_type=Fixed-point  arith_type="Signed  (2's comp)"  n_bits=16  bin_pt=15  preci_type=Single  exp_width=8  frac_width=24  rows=1  columns=1  quantization=Truncate  overflow=Wrap  period=1/8000  UseAsADC=off  ADCChannel='1'  interface=None  automatic_assignment=on  address_offset=hex2dec('00')  intf_name=''  intf_description=''  default_value=0  timing_constraint=None  locs_specified=off  LOCs={}  io_standard={}  inherit_from_input=off  hdl_port=on  dbl_ovrd=off  block_type=gatewayin
  Gateway Out{,1..3} (4 alike) : xbsIndex_r4/Gateway Out  inherit_from_input=off  hdl_port=off  rows=1  columns=1  UseAsDAC=off  DACChannel='1'  interface=None  automatic_assignment=on  address_offset=hex2dec('00')  intf_name=''  intf_description=''  timing_constraint=None  locs_specified=off  LOCs={}  io_standard={}  block_type=gatewayout
  IIR Filter : Subsystem
  IIR Filter Scope : Scope
  LPF Scope : Scope
  Low Pass Filter : Subsystem
  Mult : xbsIndex_r4/Mult  precision=User Defined  arith_type="Signed  (2's comp)"  n_bits=16  bin_pt=15  quantization=Truncate  overflow=Wrap  en=off  latency=0  use_behavioral_HDL=off  opt=Speed  use_embedded=on  optimum_pipeline=off  pipeline=on  dbl_ovrd=off  use_rpm=on  placement_style=Triangular  block_type=mult
  Sine Wave : Sin  Frequency=2*pi*fc  SampleTime=1/8000
  Output : Outport
  wires:
  Input/1 -> IIR Filter/1(Input)
  IIR Filter/1(Output) -> Gateway Out1/1, Absolute/1
  Sine Wave/1 -> Gateway In/1
  Convert/1 -> Mult/1
  Gateway In/1 -> Mult/2
  Absolute/1 -> Gateway Out2/1, Low Pass Filter/1(Input1)
  Low Pass Filter/1(Output1) -> Gateway Out3/1, Convert/1
  Gateway Out/1 -> Output/1, Final Channel Scope/1
  Mult/1 -> Gateway Out/1
  Gateway Out1/1 -> IIR Filter Scope/1
  Gateway Out2/1 -> Abs Scope/1
  Gateway Out3/1 -> LPF Scope/1

== system vocoder_model/Channel_22 ==
  Input : Inport
  Abs Scope : Scope
  Absolute : xbsIndex_r4/Absolute  precision=User Defined  arith_type="Signed  (2's comp)"  n_bits=16  bin_pt=15  quantization=Truncate  overflow=Wrap  en=off  latency=0  dbl_ovrd=off  block_type=abs
  Convert : xbsIndex_r4/Convert  gui_display_data_type=Fixed-point  arith_type="Signed  (2's comp)"  n_bits=16  bin_pt=15  float_type=Single  exp_bits=8  fraction_bits=24  quantization=Truncate  overflow=Wrap  en=off  latency=0  pipeline=off  dbl_ovrd=off  block_type=convert
  Final Channel Scope : Scope
  Gateway In : xbsIndex_r4/Gateway In  gui_display_data_type=Fixed-point  arith_type="Signed  (2's comp)"  n_bits=16  bin_pt=15  preci_type=Single  exp_width=8  frac_width=24  rows=1  columns=1  quantization=Truncate  overflow=Wrap  period=1/8000  UseAsADC=off  ADCChannel='1'  interface=None  automatic_assignment=on  address_offset=hex2dec('00')  intf_name=''  intf_description=''  default_value=0  timing_constraint=None  locs_specified=off  LOCs={}  io_standard={}  inherit_from_input=off  hdl_port=on  dbl_ovrd=off  block_type=gatewayin
  Gateway Out{,1..3} (4 alike) : xbsIndex_r4/Gateway Out  inherit_from_input=off  hdl_port=off  rows=1  columns=1  UseAsDAC=off  DACChannel='1'  interface=None  automatic_assignment=on  address_offset=hex2dec('00')  intf_name=''  intf_description=''  timing_constraint=None  locs_specified=off  LOCs={}  io_standard={}  block_type=gatewayout
  IIR Filter : Subsystem
  IIR Filter Scope : Scope
  LPF Scope : Scope
  Low Pass Filter : Subsystem
  Mult : xbsIndex_r4/Mult  precision=User Defined  arith_type="Signed  (2's comp)"  n_bits=16  bin_pt=15  quantization=Truncate  overflow=Wrap  en=off  latency=0  use_behavioral_HDL=off  opt=Speed  use_embedded=on  optimum_pipeline=off  pipeline=on  dbl_ovrd=off  use_rpm=on  placement_style=Triangular  block_type=mult
  Sine Wave : Sin  Frequency=2*pi*fc  SampleTime=1/8000
  Output : Outport
  wires:
  Input/1 -> IIR Filter/1(Input)
  IIR Filter/1(Output) -> Gateway Out1/1, Absolute/1
  Sine Wave/1 -> Gateway In/1
  Convert/1 -> Mult/1
  Gateway In/1 -> Mult/2
  Absolute/1 -> Gateway Out2/1, Low Pass Filter/1(Input1)
  Low Pass Filter/1(Output1) -> Gateway Out3/1, Convert/1
  Gateway Out/1 -> Output/1, Final Channel Scope/1
  Mult/1 -> Gateway Out/1
  Gateway Out1/1 -> IIR Filter Scope/1
  Gateway Out2/1 -> Abs Scope/1
  Gateway Out3/1 -> LPF Scope/1

== system vocoder_model/Channel_23 ==
  Input : Inport
  Abs Scope : Scope
  Absolute : xbsIndex_r4/Absolute  precision=User Defined  arith_type="Signed  (2's comp)"  n_bits=16  bin_pt=15  quantization=Truncate  overflow=Wrap  en=off  latency=0  dbl_ovrd=off  block_type=abs
  Convert : xbsIndex_r4/Convert  gui_display_data_type=Fixed-point  arith_type="Signed  (2's comp)"  n_bits=16  bin_pt=15  float_type=Single  exp_bits=8  fraction_bits=24  quantization=Truncate  overflow=Wrap  en=off  latency=0  pipeline=off  dbl_ovrd=off  block_type=convert
  Final Channel Scope : Scope
  Gateway In : xbsIndex_r4/Gateway In  gui_display_data_type=Fixed-point  arith_type="Signed  (2's comp)"  n_bits=16  bin_pt=15  preci_type=Single  exp_width=8  frac_width=24  rows=1  columns=1  quantization=Truncate  overflow=Wrap  period=1/8000  UseAsADC=off  ADCChannel='1'  interface=None  automatic_assignment=on  address_offset=hex2dec('00')  intf_name=''  intf_description=''  default_value=0  timing_constraint=None  locs_specified=off  LOCs={}  io_standard={}  inherit_from_input=off  hdl_port=on  dbl_ovrd=off  block_type=gatewayin
  Gateway Out{,1..3} (4 alike) : xbsIndex_r4/Gateway Out  inherit_from_input=off  hdl_port=off  rows=1  columns=1  UseAsDAC=off  DACChannel='1'  interface=None  automatic_assignment=on  address_offset=hex2dec('00')  intf_name=''  intf_description=''  timing_constraint=None  locs_specified=off  LOCs={}  io_standard={}  block_type=gatewayout
  IIR Filter : Subsystem
  IIR Filter Scope : Scope
  LPF Scope : Scope
  Low Pass Filter : Subsystem
  Mult : xbsIndex_r4/Mult  precision=User Defined  arith_type="Signed  (2's comp)"  n_bits=16  bin_pt=15  quantization=Truncate  overflow=Wrap  en=off  latency=0  use_behavioral_HDL=off  opt=Speed  use_embedded=on  optimum_pipeline=off  pipeline=on  dbl_ovrd=off  use_rpm=on  placement_style=Triangular  block_type=mult
  Sine Wave : Sin  Frequency=2*pi*fc  SampleTime=1/8000
  Output : Outport
  wires:
  Input/1 -> IIR Filter/1(Input)
  IIR Filter/1(Output) -> Gateway Out1/1, Absolute/1
  Sine Wave/1 -> Gateway In/1
  Convert/1 -> Mult/1
  Gateway In/1 -> Mult/2
  Absolute/1 -> Gateway Out2/1, Low Pass Filter/1(Input1)
  Low Pass Filter/1(Output1) -> Gateway Out3/1, Convert/1
  Gateway Out/1 -> Output/1, Final Channel Scope/1
  Mult/1 -> Gateway Out/1
  Gateway Out1/1 -> IIR Filter Scope/1
  Gateway Out2/1 -> Abs Scope/1
  Gateway Out3/1 -> LPF Scope/1

== system vocoder_model/Channel_24 ==
  Input : Inport
  Abs Scope : Scope
  Absolute : xbsIndex_r4/Absolute  precision=User Defined  arith_type="Signed  (2's comp)"  n_bits=16  bin_pt=15  quantization=Truncate  overflow=Wrap  en=off  latency=0  dbl_ovrd=off  block_type=abs
  Convert : xbsIndex_r4/Convert  gui_display_data_type=Fixed-point  arith_type="Signed  (2's comp)"  n_bits=16  bin_pt=15  float_type=Single  exp_bits=8  fraction_bits=24  quantization=Truncate  overflow=Wrap  en=off  latency=0  pipeline=off  dbl_ovrd=off  block_type=convert
  Final Channel Scope : Scope
  Gateway In : xbsIndex_r4/Gateway In  gui_display_data_type=Fixed-point  arith_type="Signed  (2's comp)"  n_bits=16  bin_pt=15  preci_type=Single  exp_width=8  frac_width=24  rows=1  columns=1  quantization=Truncate  overflow=Wrap  period=1/8000  UseAsADC=off  ADCChannel='1'  interface=None  automatic_assignment=on  address_offset=hex2dec('00')  intf_name=''  intf_description=''  default_value=0  timing_constraint=None  locs_specified=off  LOCs={}  io_standard={}  inherit_from_input=off  hdl_port=on  dbl_ovrd=off  block_type=gatewayin
  Gateway Out{,1..3} (4 alike) : xbsIndex_r4/Gateway Out  inherit_from_input=off  hdl_port=off  rows=1  columns=1  UseAsDAC=off  DACChannel='1'  interface=None  automatic_assignment=on  address_offset=hex2dec('00')  intf_name=''  intf_description=''  timing_constraint=None  locs_specified=off  LOCs={}  io_standard={}  block_type=gatewayout
  IIR Filter : Subsystem
  IIR Filter Scope : Scope
  LPF Scope : Scope
  Low Pass Filter : Subsystem
  Mult : xbsIndex_r4/Mult  precision=User Defined  arith_type="Signed  (2's comp)"  n_bits=16  bin_pt=15  quantization=Truncate  overflow=Wrap  en=off  latency=0  use_behavioral_HDL=off  opt=Speed  use_embedded=on  optimum_pipeline=off  pipeline=on  dbl_ovrd=off  use_rpm=on  placement_style=Triangular  block_type=mult
  Sine Wave : Sin  Frequency=2*pi*fc  SampleTime=1/8000
  Output : Outport
  wires:
  Input/1 -> IIR Filter/1(Input)
  IIR Filter/1(Output) -> Gateway Out1/1, Absolute/1
  Sine Wave/1 -> Gateway In/1
  Convert/1 -> Mult/1
  Gateway In/1 -> Mult/2
  Absolute/1 -> Gateway Out2/1, Low Pass Filter/1(Input1)
  Low Pass Filter/1(Output1) -> Gateway Out3/1, Convert/1
  Gateway Out/1 -> Output/1, Final Channel Scope/1
  Mult/1 -> Gateway Out/1
  Gateway Out1/1 -> IIR Filter Scope/1
  Gateway Out2/1 -> Abs Scope/1
  Gateway Out3/1 -> LPF Scope/1
